simulink model "Identyfikacja"  (R2023b)
settings: Solver=FixedStepDiscrete  StartTime=0.0  StopTime=tend  RelTol=1e-3  EnableMultiTasking=on
values from neighbouring files (symbols this model uses):
  Tp = 0.01    [Init_Projekt.m]
settings Model: Creator=kszygenda  LastModifiedBy=Rafał
settings SolverCC: AlgebraicLoopSolver=TrustRegion
settings DataIOCC: LimitDataPoints=on  SaveFormat=Array  SignalLoggingSaveFormat=ModelDataLogs  ReturnWorkspaceOutputs=off
settings OptimizationCC: InitFltsAndDblsToZero=on  LifeSpan=inf
settings DebuggingCC: SaveWithParameterizedLinksMsg=none  UnderspecifiedInitializationDetection=Classic  MergeDetectMultiDrivingBlocksExec=none  SignalResolutionControl=TryResolveAllWithWarning  SolverPrmCheckMsg=warning  MultiTaskDSMMsg=warning  MultiTaskCondExecSysMsg=none  FcnCallInpInsideContextMsg=warning  UnconnectedInputMsg=warning  UnconnectedOutputMsg=warning  UnconnectedLineMsg=warning  SFUnexpectedBacktrackingDiag=warning  SFNoUnconditionalDefaultTransitionDiag=warning  SFExecutionAtInitializationDiag=none  ArithmeticOperatorsInVariantConditions=warning
settings HardwareCC: ProdBitPerPointer=32  ProdBitPerSizeT=32  ProdBitPerPtrDiffT=32  ProdLargestAtomicFloat=None  ProdIntDivRoundTo=Undefined  ProdEndianess=Unspecified  ProdWordSize=32  ProdHWDeviceType=32-bit Generic
settings ModelReferenceCC: PropagateSignalLabelsOutOfModel=off
settings CodeAppCC: StateflowObjectComments=on
settings GRTTargetCC: TargetFcnLib=ansi_tfl_tmw.mat  TargetLangStandard=C89/C90 (ANSI)  CombineOutputUpdateFcns=off  GRTInterface=on
settings ConfigComp: CovMetricSettings=dw  CovSaveCumulativeToWorkspaceVar=on  CovSaveSingleToWorkspaceVar=on

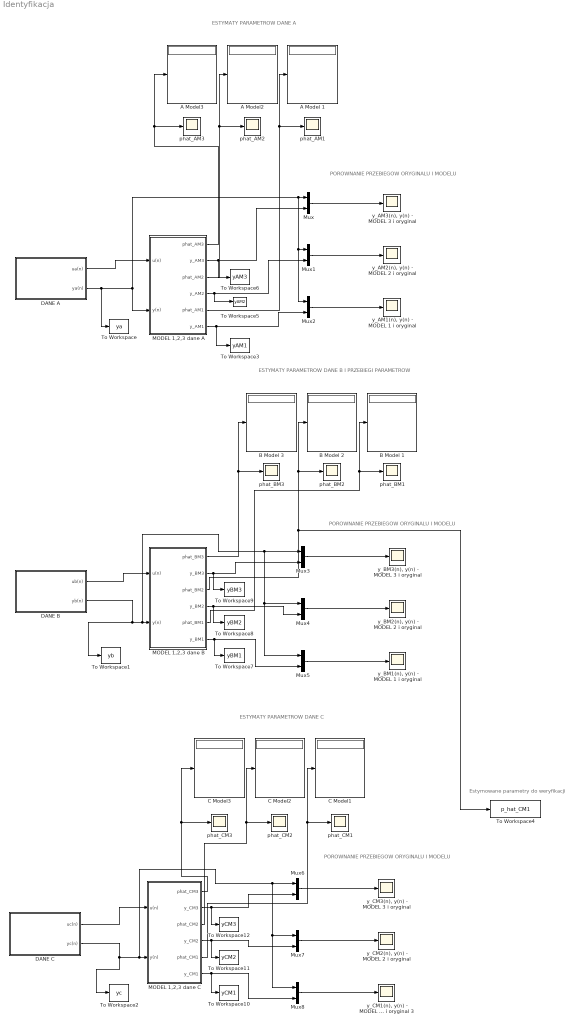
== system Identyfikacja ==
  note: Estymowane parametry do weryfikacji
  note: ESTYMATY PARAMETROW DANE A
  note: ESTYMATY PARAMETROW DANE B I PRZEBIEGI PARAMETROW
  note: ESTYMATY PARAMETROW DANE C
  note: POROWNANIE PRZEBIEGOW ORYGINALU I MODELU
  note: POROWNANIE PRZEBIEGOW ORYGINALU I MODELU
  note: POROWNANIE PRZEBIEGOW ORYGINALU I MODELU
  A Model 1 : Display
  A Model2 : Display
  A Model3 : Display
  B Model 1 : Display
  B Model 2 : Display
  B Model 3 : Display
  C Model1 : Display
  C Model2 : Display
  C Model3 : Display
  DANE A : Subsystem
  DANE B : Subsystem
  DANE C : Subsystem
  MODEL 1,2,3 dane A : Subsystem
  MODEL 1,2,3 dane B : Subsystem
  MODEL 1,2,3 dane C : Subsystem
  Mux{,1..8} (9 alike) : Mux  Inputs=2
  To Workspace : ToWorkspace  VariableName=ya  SampleTime=Tp
      settings: Save2DSignal=2-D array (concatenate along first dimension)
  To Workspace1 : ToWorkspace  VariableName=yb  SampleTime=Tp
      settings: Save2DSignal=2-D array (concatenate along first dimension)
  To Workspace10 : ToWorkspace  VariableName=yCM1  SampleTime=Tp
      settings: Save2DSignal=2-D array (concatenate along first dimension)
  To Workspace11 : ToWorkspace  VariableName=yCM2  SampleTime=Tp
      settings: Save2DSignal=2-D array (concatenate along first dimension)
  To Workspace12 : ToWorkspace  VariableName=yCM3  SampleTime=Tp
      settings: Save2DSignal=2-D array (concatenate along first dimension)
  To Workspace2 : ToWorkspace  VariableName=yc  SampleTime=Tp
      settings: Save2DSignal=2-D array (concatenate along first dimension)
  To Workspace3 : ToWorkspace  VariableName=yAM1  SampleTime=Tp
      settings: Save2DSignal=2-D array (concatenate along first dimension)
  To Workspace4 : ToWorkspace  VariableName=p_hat_CM1  SampleTime=Tp
      settings: Save2DSignal=2-D array (concatenate along first dimension)
  To Workspace5 : ToWorkspace  VariableName=yAM2  SampleTime=Tp
      settings: Save2DSignal=2-D array (concatenate along first dimension)
  To Workspace6 : ToWorkspace  VariableName=yAM3  SampleTime=Tp
      settings: Save2DSignal=2-D array (concatenate along first dimension)
  To Workspace7 : ToWorkspace  VariableName=yBM1  SampleTime=Tp
      settings: Save2DSignal=2-D array (concatenate along first dimension)
  To Workspace8 : ToWorkspace  VariableName=yBM2  SampleTime=Tp
      settings: Save2DSignal=2-D array (concatenate along first dimension)
  To Workspace9 : ToWorkspace  VariableName=yBM3  SampleTime=Tp
      settings: Save2DSignal=2-D array (concatenate along first dimension)
  phat_AM1 : Scope
  phat_AM2 : Scope
  phat_AM3 : Scope
  phat_BM1 : Scope
  phat_BM2 : Scope
  phat_BM3 : Scope
  phat_CM1 : Scope
  phat_CM2 : Scope
  phat_CM3 : Scope
  "y_AM1(n), y(n) - MODEL 1 i oryginal" : Scope
  "y_AM2(n), y(n) - MODEL 2 i oryginal " : Scope
  "y_AM3(n), y(n) - MODEL 3 i oryginal " : Scope
  "y_BM1(n), y(n) - MODEL 1 i oryginal" : Scope
  "y_BM2(n), y(n) - MODEL 2 i oryginal" : Scope
  "y_BM3(n), y(n) - MODEL 3 i oryginal" : Scope
  "y_CM1(n), y(n) - MODEL 1 i oryginal 3" : Scope
  "y_CM2(n), y(n) - MODEL 2 i oryginal" : Scope
  "y_CM3(n), y(n) - MODEL 3 i oryginal" : Scope
  wires:
  DANE C/1(uc(n)) -> MODEL 1,2,3 dane C/1(u(n))
  DANE C/2(yc(n)) -> To Workspace2/1, Mux6/1, Mux7/1, Mux8/1, MODEL 1,2,3 dane C/2(y(n))
  DANE B/1(ub(n)) -> MODEL 1,2,3 dane B/1(u(n))
  DANE B/2(yb(n)) -> To Workspace1/1, Mux3/1, Mux5/1, Mux4/1, MODEL 1,2,3 dane B/2(y(n))
  DANE A/1(ua(n)) -> MODEL 1,2,3 dane A/1(u(n))
  DANE A/2(ya(n)) -> To Workspace/1, Mux1/1, Mux2/1, Mux/1, MODEL 1,2,3 dane A/2(y(n))
  Mux/1 -> "y_AM3(n), y(n) - MODEL 3 i oryginal "/1
  MODEL 1,2,3 dane A/2(y_AM3) -> To Workspace6/1, Mux/2
  Mux1/1 -> "y_AM2(n), y(n) - MODEL 2 i oryginal "/1
  Mux2/1 -> "y_AM1(n), y(n) - MODEL 1 i oryginal"/1
  Mux3/1 -> "y_BM3(n), y(n) - MODEL 3 i oryginal"/1
  Mux5/1 -> "y_BM1(n), y(n) - MODEL 1 i oryginal"/1
  Mux4/1 -> "y_BM2(n), y(n) - MODEL 2 i oryginal"/1
  Mux6/1 -> "y_CM3(n), y(n) - MODEL 3 i oryginal"/1
  Mux8/1 -> "y_CM1(n), y(n) - MODEL 1 i oryginal 3"/1
  Mux7/1 -> "y_CM2(n), y(n) - MODEL 2 i oryginal"/1
  MODEL 1,2,3 dane A/4(y_AM2) -> Mux1/2, To Workspace5/1
  MODEL 1,2,3 dane A/6(y_AM1) -> Mux2/2, To Workspace3/1
  MODEL 1,2,3 dane C/2(y_CM3) -> To Workspace12/1, Mux6/2
  MODEL 1,2,3 dane C/4(y_CM2) -> To Workspace11/1, Mux7/2
  MODEL 1,2,3 dane C/6(y_CM1) -> To Workspace10/1, Mux8/2
  MODEL 1,2,3 dane B/2(y_BM3) -> To Workspace9/1, Mux3/2
  MODEL 1,2,3 dane B/4(y_BM2) -> To Workspace8/1, Mux4/2
  MODEL 1,2,3 dane B/6(y_BM1) -> To Workspace7/1, Mux5/2
  MODEL 1,2,3 dane A/1(phat_AM3) -> phat_AM3/1, A Model3/1
  MODEL 1,2,3 dane A/3(phat_AM2) -> phat_AM2/1, A Model2/1
  MODEL 1,2,3 dane A/5(phat_AM1) -> A Model 1/1, phat_AM1/1
  MODEL 1,2,3 dane B/1(phat_BM3) -> phat_BM3/1, B Model 3/1
  MODEL 1,2,3 dane B/3(phat_BM2) -> phat_BM2/1, B Model 2/1, To Workspace4/1
  MODEL 1,2,3 dane B/5(phat_BM1) -> B Model 1/1, phat_BM1/1
  MODEL 1,2,3 dane C/1(phat_CM3) -> phat_CM3/1, C Model3/1
  MODEL 1,2,3 dane C/3(phat_CM2) -> phat_CM2/1, C Model2/1
  MODEL 1,2,3 dane C/5(phat_CM1) -> phat_CM1/1, C Model1/1

== system Identyfikacja/DANE A ==
  Demux : Demux  Outputs=2
  From Workspace : FromWorkspace  VariableName=to_simA  SampleTime=Tp
  ua(n) : Outport
  ya(n) : Outport  Port=2
  wires:
  Demux/1 -> ua(n)/1
  From Workspace/1 -> Demux/1
  Demux/2 -> ya(n)/1

== system Identyfikacja/DANE B ==
  Demux : Demux  Outputs=2
  From Workspace : FromWorkspace  VariableName=to_simB  SampleTime=Tp
  ub(n) : Outport
  yb(n) : Outport  Port=2
  wires:
  Demux/1 -> ub(n)/1
  From Workspace/1 -> Demux/1
  Demux/2 -> yb(n)/1

== system Identyfikacja/DANE C ==
  Demux : Demux  Outputs=2
  From Workspace : FromWorkspace  VariableName=to_simC  SampleTime=Tp
  uc(n) : Outport
  yc(n) : Outport  Port=2
  wires:
  Demux/1 -> uc(n)/1
  From Workspace/1 -> Demux/1
  Demux/2 -> yc(n)/1

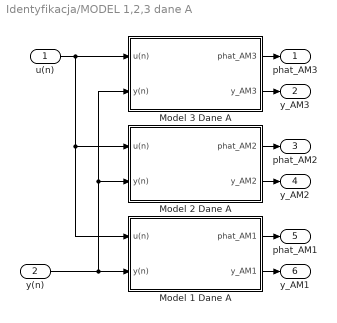
== system Identyfikacja/MODEL 1,2,3 dane A ==
  u(n) : Inport
  y(n) : Inport  Port=2
  Model 1 Dane A : Subsystem
  Model 2 Dane A : Subsystem
  Model 3 Dane A : Subsystem
  phat_AM3 : Outport
  y_AM3 : Outport  Port=2
  phat_AM2 : Outport  Port=3
  y_AM2 : Outport  Port=4
  phat_AM1 : Outport  Port=5
  y_AM1 : Outport  Port=6
  wires:
  Model 1 Dane A/1(phat_AM1) -> phat_AM1/1
  u(n)/1 -> Model 3 Dane A/1(u(n)), Model 2 Dane A/1(u(n)), Model 1 Dane A/1(u(n))
  Model 1 Dane A/2(y_AM1) -> y_AM1/1
  y(n)/1 -> Model 2 Dane A/2(y(n)), Model 3 Dane A/2(y(n)), Model 1 Dane A/2(y(n))
  Model 3 Dane A/1(phat_AM3) -> phat_AM3/1
  Model 3 Dane A/2(y_AM3) -> y_AM3/1
  Model 2 Dane A/2(y_AM2) -> y_AM2/1
  Model 2 Dane A/1(phat_AM2) -> phat_AM2/1

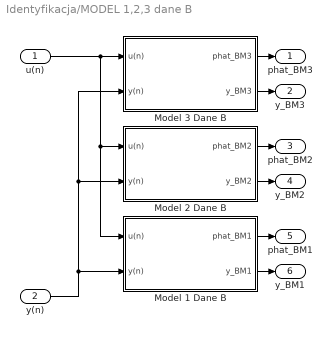
== system Identyfikacja/MODEL 1,2,3 dane B ==
  u(n) : Inport
  y(n) : Inport  Port=2
  Model 1 Dane B : Subsystem
  Model 2 Dane B : Subsystem
  Model 3 Dane B : Subsystem
  phat_BM3 : Outport
  y_BM3 : Outport  Port=2
  phat_BM2 : Outport  Port=3
  y_BM2 : Outport  Port=4
  phat_BM1 : Outport  Port=5
  y_BM1 : Outport  Port=6
  wires:
  Model 3 Dane B/1(phat_BM3) -> phat_BM3/1
  u(n)/1 -> Model 3 Dane B/1(u(n)), Model 2 Dane B/1(u(n)), Model 1 Dane B/1(u(n))
  Model 1 Dane B/1(phat_BM1) -> phat_BM1/1
  Model 3 Dane B/2(y_BM3) -> y_BM3/1
  y(n)/1 -> Model 1 Dane B/2(y(n)), Model 2 Dane B/2(y(n)), Model 3 Dane B/2(y(n))
  Model 2 Dane B/2(y_BM2) -> y_BM2/1
  Model 1 Dane B/2(y_BM1) -> y_BM1/1
  Model 2 Dane B/1(phat_BM2) -> phat_BM2/1

== system Identyfikacja/MODEL 1,2,3 dane C ==
  u(n) : Inport
  y(n) : Inport  Port=2
  Model 1 Dane C : Subsystem
  Model 2 Dane C : Subsystem
  Model 3 Dane C : Subsystem
  phat_CM3 : Outport
  y_CM3 : Outport  Port=2
  phat_CM2 : Outport  Port=3
  y_CM2 : Outport  Port=4
  phat_CM1 : Outport  Port=5
  y_CM1 : Outport  Port=6
  wires:
  u(n)/1 -> Model 3 Dane C/1(u(n)), Model 2 Dane C/1(u(n)), Model 1 Dane C/1(u(n))
  Model 2 Dane C/2(y_CM2) -> y_CM2/1
  Model 3 Dane C/2(y_CM3) -> y_CM3/1
  Model 3 Dane C/1(phat_CM3) -> phat_CM3/1
  Model 1 Dane C/2(y_CM1) -> y_CM1/1
  Model 2 Dane C/1(phat_CM2) -> phat_CM2/1
  Model 1 Dane C/1(phat_CM1) -> phat_CM1/1
  y(n)/1 -> Model 1 Dane C/2(y(n)), Model 2 Dane C/2(y(n)), Model 3 Dane C/2(y(n))

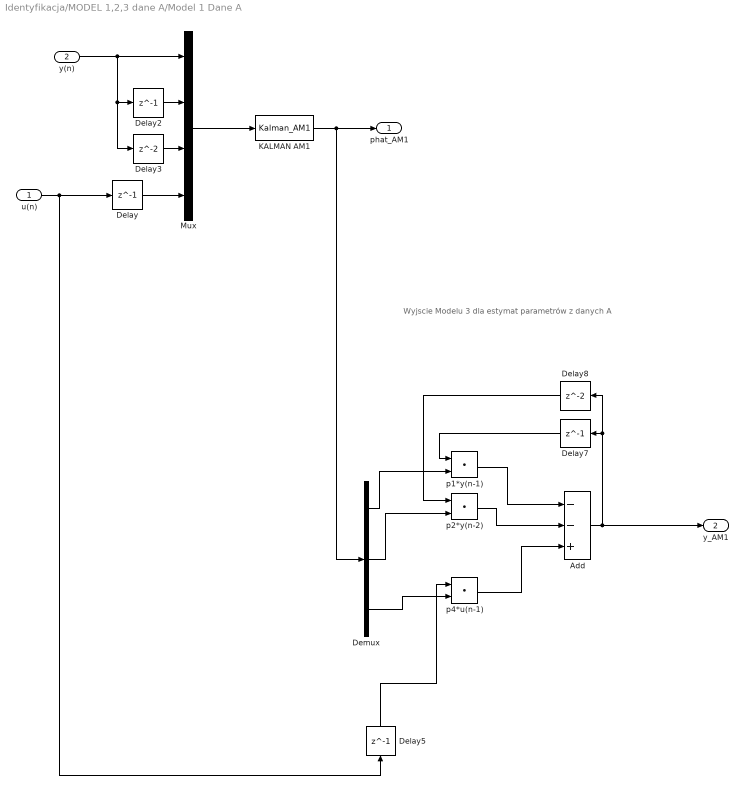
== system Identyfikacja/MODEL 1,2,3 dane A/Model 1 Dane A ==
  note: Wyjscie Modelu 3 dla estymat parametrów z danych A
  u(n) : Inport
  y(n) : Inport  Port=2
  Add : Sum  Inputs=--+
  Delay{,2,5,7} (4 alike) : Delay  DelayLength=1  InitialCondition=0  SampleTime=Tp
  Delay3 : Delay  InitialCondition=0  SampleTime=Tp
  Delay8 : Delay  InitialCondition=0  SampleTime=Tp
  Demux : Demux  Outputs=3
  KALMAN AM1 : MATLABFcn  MATLABFcn=Kalman_AM1  OutputDimensions=3
  Mux : Mux
  p1*y(n-1) : DotProduct  OutDataTypeStr=Inherit: Inherit via internal rule
  p2*y(n-2) : DotProduct  OutDataTypeStr=Inherit: Inherit via internal rule
  p4*u(n-1) : DotProduct  OutDataTypeStr=Inherit: Inherit via internal rule
  phat_AM1 : Outport
  y_AM1 : Outport  Port=2
  wires:
  y(n)/1 -> Mux/1, Delay3/1, Delay2/1
  Mux/1 -> KALMAN AM1/1
  KALMAN AM1/1 -> Demux/1, phat_AM1/1
  p1*y(n-1)/1 -> Add/1
  Demux/2 -> p2*y(n-2)/2
  Delay8/1 -> p2*y(n-2)/1
  p2*y(n-2)/1 -> Add/2
  Delay5/1 -> p4*u(n-1)/1
  Delay7/1 -> p1*y(n-1)/1
  Demux/1 -> p1*y(n-1)/2
  u(n)/1 -> Delay/1, Delay5/1
  Demux/3 -> p4*u(n-1)/2
  Add/1 -> y_AM1/1, Delay8/1, Delay7/1
  p4*u(n-1)/1 -> Add/3
  Delay2/1 -> Mux/2
  Delay3/1 -> Mux/3
  Delay/1 -> Mux/4

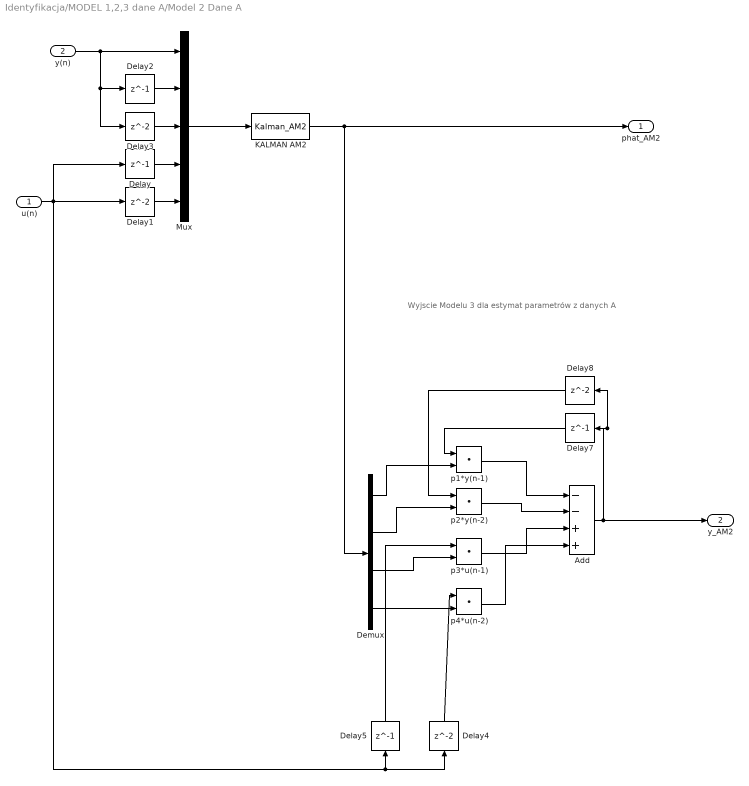
== system Identyfikacja/MODEL 1,2,3 dane A/Model 2 Dane A ==
  note: Wyjscie Modelu 3 dla estymat parametrów z danych A
  u(n) : Inport
  y(n) : Inport  Port=2
  Add : Sum  Inputs=--++
  Delay{,2,5,7} (4 alike) : Delay  DelayLength=1  InitialCondition=0  SampleTime=Tp
  Delay{1,3..4,8} (4 alike) : Delay  InitialCondition=0  SampleTime=Tp
  Demux : Demux
  KALMAN AM2 : MATLABFcn  MATLABFcn=Kalman_AM2  OutputDimensions=4
  Mux : Mux  Inputs=5
  p1*y(n-1) : DotProduct  OutDataTypeStr=Inherit: Inherit via internal rule
  p2*y(n-2) : DotProduct  OutDataTypeStr=Inherit: Inherit via internal rule
  p3*u(n-1) : DotProduct  OutDataTypeStr=Inherit: Inherit via internal rule
  p4*u(n-2) : DotProduct  OutDataTypeStr=Inherit: Inherit via internal rule
  phat_AM2 : Outport
  y_AM2 : Outport  Port=2
  wires:
  y(n)/1 -> Mux/1, Delay3/1, Delay2/1
  Delay5/1 -> p3*u(n-1)/1
  p1*y(n-1)/1 -> Add/1
  Demux/2 -> p2*y(n-2)/2
  p2*y(n-2)/1 -> Add/2
  Delay7/1 -> p1*y(n-1)/1
  Delay4/1 -> p4*u(n-2)/1
  Delay/1 -> Mux/4
  KALMAN AM2/1 -> Demux/1, phat_AM2/1
  Demux/4 -> p4*u(n-2)/2
  Add/1 -> Delay8/1, Delay7/1, y_AM2/1
  Delay8/1 -> p2*y(n-2)/1
  Delay3/1 -> Mux/3
  u(n)/1 -> Delay/1, Delay1/1, Delay4/1, Delay5/1
  Delay2/1 -> Mux/2
  Demux/3 -> p3*u(n-1)/2
  p4*u(n-2)/1 -> Add/4
  Delay1/1 -> Mux/5
  p3*u(n-1)/1 -> Add/3
  Mux/1 -> KALMAN AM2/1
  Demux/1 -> p1*y(n-1)/2

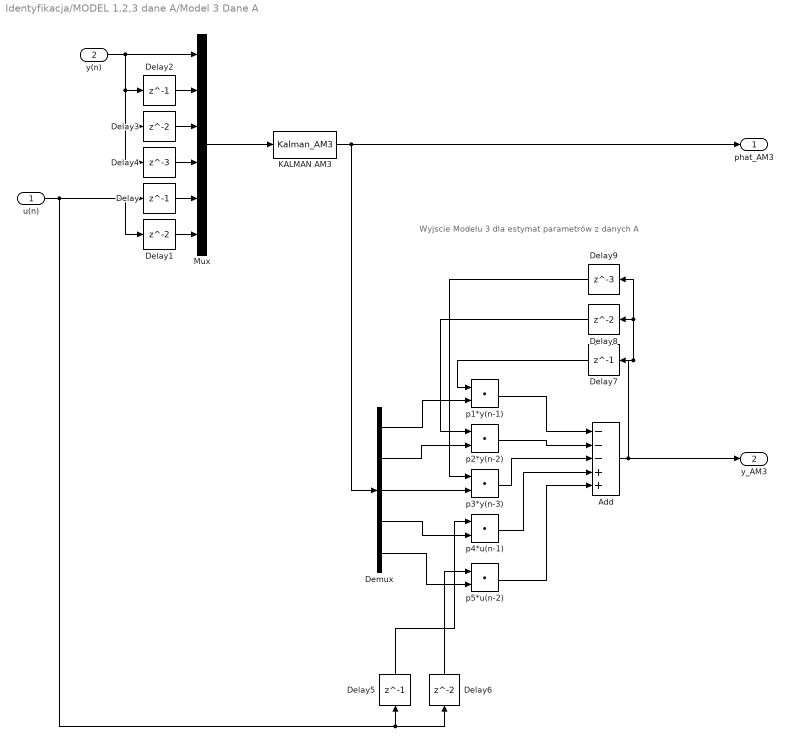
== system Identyfikacja/MODEL 1,2,3 dane A/Model 3 Dane A ==
  note: Wyjscie Modelu 3 dla estymat parametrów z danych A
  u(n) : Inport
  y(n) : Inport  Port=2
  Add : Sum  Inputs=---++
  Delay{,2,5,7} (4 alike) : Delay  DelayLength=1  InitialCondition=0  SampleTime=Tp
  Delay{1,3,6,8} (4 alike) : Delay  InitialCondition=0  SampleTime=Tp
  Delay4 : Delay  DelayLength=3  InitialCondition=0  SampleTime=Tp
  Delay9 : Delay  DelayLength=3  InitialCondition=0  SampleTime=Tp
  Demux : Demux  Outputs=5
  KALMAN AM3 : MATLABFcn  MATLABFcn=Kalman_AM3  OutputDimensions=5
  Mux : Mux  Inputs=6
  p1*y(n-1) : DotProduct  OutDataTypeStr=Inherit: Inherit via internal rule
  p2*y(n-2) : DotProduct  OutDataTypeStr=Inherit: Inherit via internal rule
  p3*y(n-3) : DotProduct  OutDataTypeStr=Inherit: Inherit via internal rule
  p4*u(n-1) : DotProduct  OutDataTypeStr=Inherit: Inherit via internal rule
  p5*u(n-2) : DotProduct  OutDataTypeStr=Inherit: Inherit via internal rule
  phat_AM3 : Outport
  y_AM3 : Outport  Port=2
  wires:
  KALMAN AM3/1 -> Demux/1, phat_AM3/1
  y(n)/1 -> Mux/1, Delay4/1, Delay3/1, Delay2/1
  Mux/1 -> KALMAN AM3/1
  Add/1 -> Delay9/1, Delay8/1, Delay7/1, y_AM3/1
  Demux/1 -> p1*y(n-1)/2
  Demux/2 -> p2*y(n-2)/2
  Demux/5 -> p5*u(n-2)/2
  Demux/4 -> p4*u(n-1)/2
  Demux/3 -> p3*y(n-3)/2
  u(n)/1 -> Delay6/1, Delay5/1, Delay1/1, Delay/1
  Delay5/1 -> p4*u(n-1)/1
  Delay6/1 -> p5*u(n-2)/1
  p5*u(n-2)/1 -> Add/5
  p4*u(n-1)/1 -> Add/4
  p3*y(n-3)/1 -> Add/3
  p2*y(n-2)/1 -> Add/2
  p1*y(n-1)/1 -> Add/1
  Delay7/1 -> p1*y(n-1)/1
  Delay8/1 -> p2*y(n-2)/1
  Delay9/1 -> p3*y(n-3)/1
  Delay4/1 -> Mux/4
  Delay3/1 -> Mux/3
  Delay2/1 -> Mux/2
  Delay1/1 -> Mux/6
  Delay/1 -> Mux/5

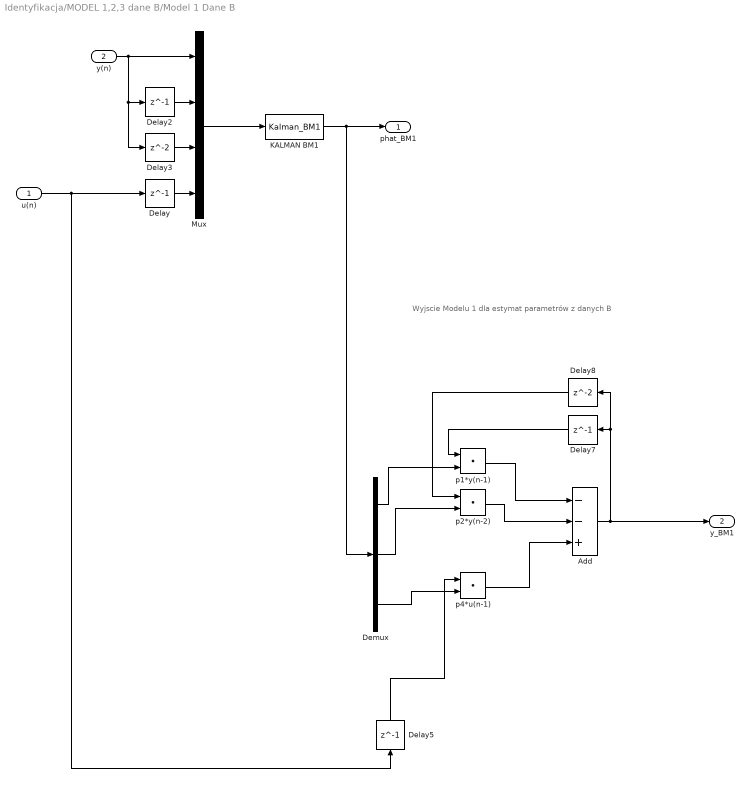
== system Identyfikacja/MODEL 1,2,3 dane B/Model 1 Dane B ==
  note: Wyjscie Modelu 1 dla estymat parametrów z danych B
  u(n) : Inport
  y(n) : Inport  Port=2
  Add : Sum  Inputs=--+
  Delay{,2,5,7} (4 alike) : Delay  DelayLength=1  InitialCondition=0  SampleTime=Tp
  Delay3 : Delay  InitialCondition=0  SampleTime=Tp
  Delay8 : Delay  InitialCondition=0  SampleTime=Tp
  Demux : Demux  Outputs=3
  KALMAN BM1 : MATLABFcn  MATLABFcn=Kalman_BM1  OutputDimensions=3
  Mux : Mux
  p1*y(n-1) : DotProduct  OutDataTypeStr=Inherit: Inherit via internal rule
  p2*y(n-2) : DotProduct  OutDataTypeStr=Inherit: Inherit via internal rule
  p4*u(n-1) : DotProduct  OutDataTypeStr=Inherit: Inherit via internal rule
  phat_BM1 : Outport
  y_BM1 : Outport  Port=2
  wires:
  y(n)/1 -> Mux/1, Delay3/1, Delay2/1
  Mux/1 -> KALMAN BM1/1
  KALMAN BM1/1 -> Demux/1, phat_BM1/1
  p1*y(n-1)/1 -> Add/1
  Demux/2 -> p2*y(n-2)/2
  Delay8/1 -> p2*y(n-2)/1
  p2*y(n-2)/1 -> Add/2
  Delay5/1 -> p4*u(n-1)/1
  Delay7/1 -> p1*y(n-1)/1
  Demux/1 -> p1*y(n-1)/2
  u(n)/1 -> Delay5/1, Delay/1
  Demux/3 -> p4*u(n-1)/2
  Add/1 -> y_BM1/1, Delay8/1, Delay7/1
  p4*u(n-1)/1 -> Add/3
  Delay3/1 -> Mux/3
  Delay2/1 -> Mux/2
  Delay/1 -> Mux/4

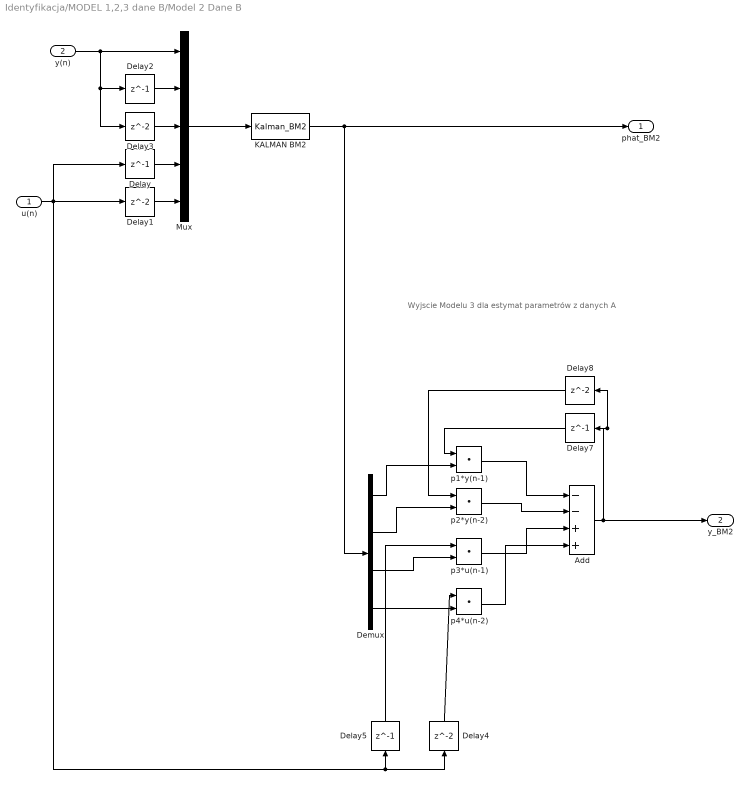
== system Identyfikacja/MODEL 1,2,3 dane B/Model 2 Dane B ==
  note: Wyjscie Modelu 3 dla estymat parametrów z danych A
  u(n) : Inport
  y(n) : Inport  Port=2
  Add : Sum  Inputs=--++
  Delay{,2,5,7} (4 alike) : Delay  DelayLength=1  InitialCondition=0  SampleTime=Tp
  Delay{1,3..4,8} (4 alike) : Delay  InitialCondition=0  SampleTime=Tp
  Demux : Demux
  KALMAN BM2 : MATLABFcn  MATLABFcn=Kalman_BM2  OutputDimensions=4
  Mux : Mux  Inputs=5
  p1*y(n-1) : DotProduct  OutDataTypeStr=Inherit: Inherit via internal rule
  p2*y(n-2) : DotProduct  OutDataTypeStr=Inherit: Inherit via internal rule
  p3*u(n-1) : DotProduct  OutDataTypeStr=Inherit: Inherit via internal rule
  p4*u(n-2) : DotProduct  OutDataTypeStr=Inherit: Inherit via internal rule
  phat_BM2 : Outport
  y_BM2 : Outport  Port=2
  wires:
  y(n)/1 -> Mux/1, Delay3/1, Delay2/1
  Mux/1 -> KALMAN BM2/1
  u(n)/1 -> Delay/1, Delay1/1, Delay4/1, Delay5/1
  Delay8/1 -> p2*y(n-2)/1
  Add/1 -> Delay8/1, Delay7/1, y_BM2/1
  Demux/1 -> p1*y(n-1)/2
  Delay7/1 -> p1*y(n-1)/1
  Delay5/1 -> p3*u(n-1)/1
  KALMAN BM2/1 -> Demux/1, phat_BM2/1
  p2*y(n-2)/1 -> Add/2
  Demux/2 -> p2*y(n-2)/2
  p1*y(n-1)/1 -> Add/1
  Delay3/1 -> Mux/3
  Delay2/1 -> Mux/2
  Delay/1 -> Mux/4
  Delay1/1 -> Mux/5
  Demux/3 -> p3*u(n-1)/2
  p3*u(n-1)/1 -> Add/3
  Delay4/1 -> p4*u(n-2)/1
  Demux/4 -> p4*u(n-2)/2
  p4*u(n-2)/1 -> Add/4

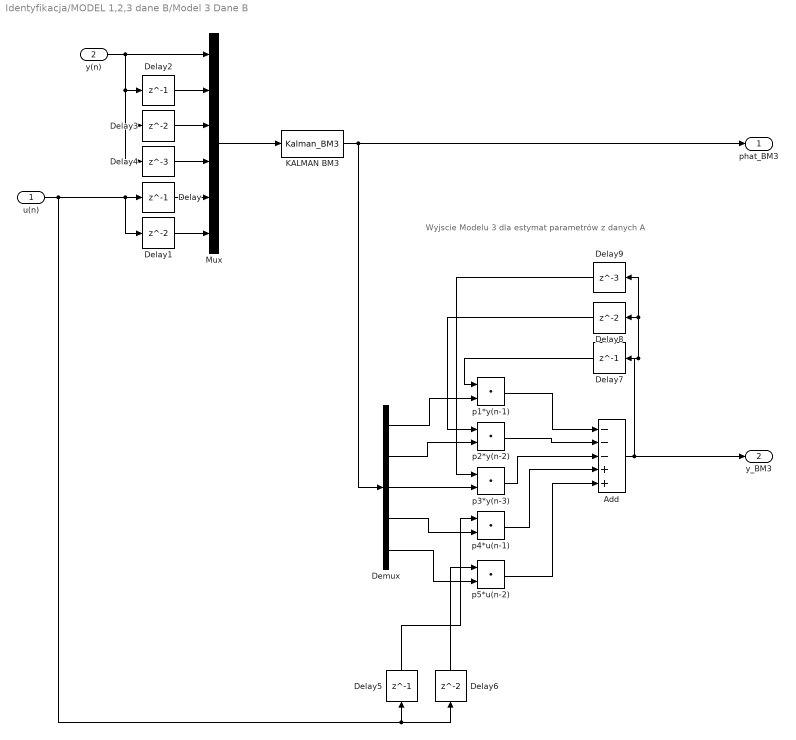
== system Identyfikacja/MODEL 1,2,3 dane B/Model 3 Dane B ==
  note: Wyjscie Modelu 3 dla estymat parametrów z danych A
  u(n) : Inport
  y(n) : Inport  Port=2
  Add : Sum  Inputs=---++
  Delay{,2,5,7} (4 alike) : Delay  DelayLength=1  InitialCondition=0  SampleTime=Tp
  Delay{1,3,6,8} (4 alike) : Delay  InitialCondition=0  SampleTime=Tp
  Delay4 : Delay  DelayLength=3  InitialCondition=0  SampleTime=Tp
  Delay9 : Delay  DelayLength=3  InitialCondition=0  SampleTime=Tp
  Demux : Demux  Outputs=5
  KALMAN BM3 : MATLABFcn  MATLABFcn=Kalman_BM3  OutputDimensions=5
  Mux : Mux  Inputs=6
  p1*y(n-1) : DotProduct  OutDataTypeStr=Inherit: Inherit via internal rule
  p2*y(n-2) : DotProduct  OutDataTypeStr=Inherit: Inherit via internal rule
  p3*y(n-3) : DotProduct  OutDataTypeStr=Inherit: Inherit via internal rule
  p4*u(n-1) : DotProduct  OutDataTypeStr=Inherit: Inherit via internal rule
  p5*u(n-2) : DotProduct  OutDataTypeStr=Inherit: Inherit via internal rule
  phat_BM3 : Outport
  y_BM3 : Outport  Port=2
  wires:
  KALMAN BM3/1 -> Demux/1, phat_BM3/1
  y(n)/1 -> Mux/1, Delay4/1, Delay3/1, Delay2/1
  Mux/1 -> KALMAN BM3/1
  Add/1 -> Delay9/1, Delay8/1, Delay7/1, y_BM3/1
  Demux/1 -> p1*y(n-1)/2
  Demux/2 -> p2*y(n-2)/2
  Demux/5 -> p5*u(n-2)/2
  Demux/4 -> p4*u(n-1)/2
  Demux/3 -> p3*y(n-3)/2
  u(n)/1 -> Delay6/1, Delay5/1, Delay1/1, Delay/1
  Delay5/1 -> p4*u(n-1)/1
  Delay6/1 -> p5*u(n-2)/1
  p5*u(n-2)/1 -> Add/5
  p4*u(n-1)/1 -> Add/4
  p3*y(n-3)/1 -> Add/3
  p2*y(n-2)/1 -> Add/2
  p1*y(n-1)/1 -> Add/1
  Delay7/1 -> p1*y(n-1)/1
  Delay8/1 -> p2*y(n-2)/1
  Delay9/1 -> p3*y(n-3)/1
  Delay4/1 -> Mux/4
  Delay3/1 -> Mux/3
  Delay2/1 -> Mux/2
  Delay/1 -> Mux/5
  Delay1/1 -> Mux/6

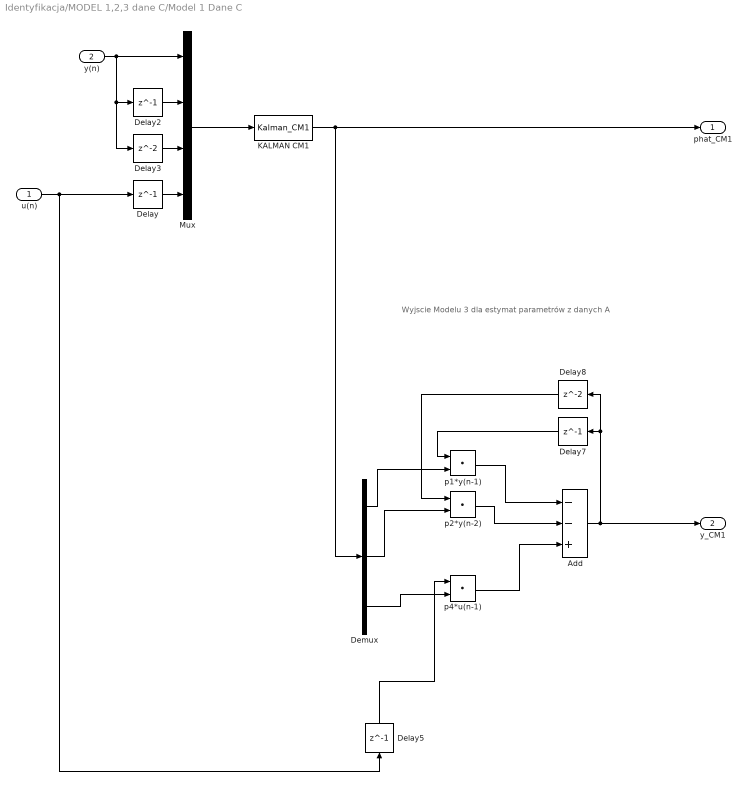
== system Identyfikacja/MODEL 1,2,3 dane C/Model 1 Dane C ==
  note: Wyjscie Modelu 3 dla estymat parametrów z danych A
  u(n) : Inport
  y(n) : Inport  Port=2
  Add : Sum  Inputs=--+
  Delay{,2,5,7} (4 alike) : Delay  DelayLength=1  InitialCondition=0  SampleTime=Tp
  Delay3 : Delay  InitialCondition=0  SampleTime=Tp
  Delay8 : Delay  InitialCondition=0  SampleTime=Tp
  Demux : Demux  Outputs=3
  KALMAN CM1 : MATLABFcn  MATLABFcn=Kalman_CM1  OutputDimensions=3
  Mux : Mux
  p1*y(n-1) : DotProduct  OutDataTypeStr=Inherit: Inherit via internal rule
  p2*y(n-2) : DotProduct  OutDataTypeStr=Inherit: Inherit via internal rule
  p4*u(n-1) : DotProduct  OutDataTypeStr=Inherit: Inherit via internal rule
  phat_CM1 : Outport
  y_CM1 : Outport  Port=2
  wires:
  y(n)/1 -> Mux/1, Delay3/1, Delay2/1
  Mux/1 -> KALMAN CM1/1
  KALMAN CM1/1 -> Demux/1, phat_CM1/1
  p1*y(n-1)/1 -> Add/1
  Demux/2 -> p2*y(n-2)/2
  Delay8/1 -> p2*y(n-2)/1
  p2*y(n-2)/1 -> Add/2
  Delay5/1 -> p4*u(n-1)/1
  Delay7/1 -> p1*y(n-1)/1
  Demux/1 -> p1*y(n-1)/2
  u(n)/1 -> Delay5/1, Delay/1
  Demux/3 -> p4*u(n-1)/2
  Add/1 -> y_CM1/1, Delay8/1, Delay7/1
  p4*u(n-1)/1 -> Add/3
  Delay3/1 -> Mux/3
  Delay2/1 -> Mux/2
  Delay/1 -> Mux/4

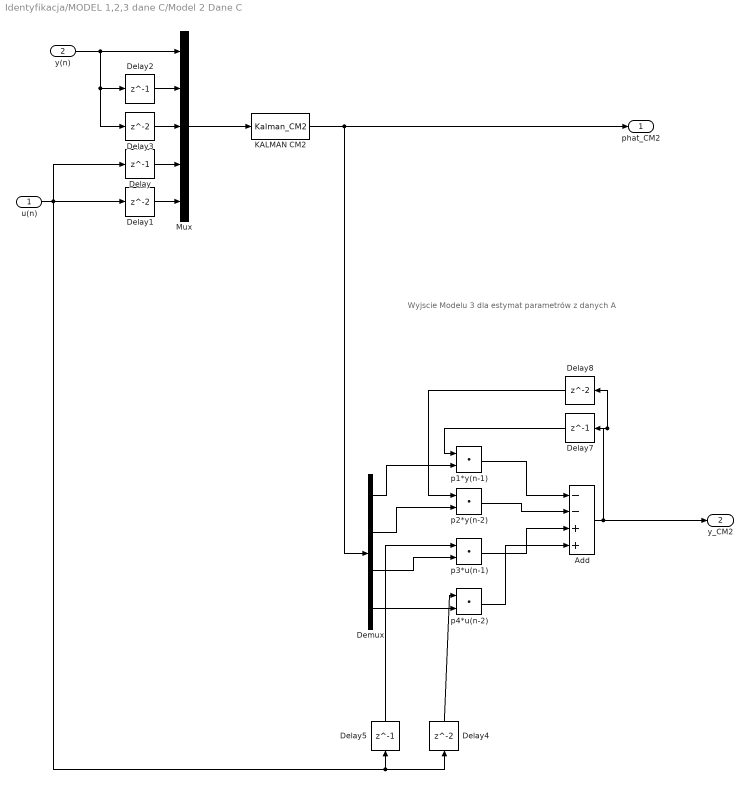
== system Identyfikacja/MODEL 1,2,3 dane C/Model 2 Dane C ==
  note: Wyjscie Modelu 3 dla estymat parametrów z danych A
  u(n) : Inport
  y(n) : Inport  Port=2
  Add : Sum  Inputs=--++
  Delay{,2,5,7} (4 alike) : Delay  DelayLength=1  InitialCondition=0  SampleTime=Tp
  Delay{1,3..4,8} (4 alike) : Delay  InitialCondition=0  SampleTime=Tp
  Demux : Demux
  KALMAN CM2 : MATLABFcn  MATLABFcn=Kalman_CM2  OutputDimensions=4
  Mux : Mux  Inputs=5
  p1*y(n-1) : DotProduct  OutDataTypeStr=Inherit: Inherit via internal rule
  p2*y(n-2) : DotProduct  OutDataTypeStr=Inherit: Inherit via internal rule
  p3*u(n-1) : DotProduct  OutDataTypeStr=Inherit: Inherit via internal rule
  p4*u(n-2) : DotProduct  OutDataTypeStr=Inherit: Inherit via internal rule
  phat_CM2 : Outport
  y_CM2 : Outport  Port=2
  wires:
  y(n)/1 -> Mux/1, Delay3/1, Delay2/1
  Delay5/1 -> p3*u(n-1)/1
  p1*y(n-1)/1 -> Add/1
  Demux/2 -> p2*y(n-2)/2
  p2*y(n-2)/1 -> Add/2
  Delay7/1 -> p1*y(n-1)/1
  Delay4/1 -> p4*u(n-2)/1
  Delay/1 -> Mux/4
  KALMAN CM2/1 -> Demux/1, phat_CM2/1
  Demux/4 -> p4*u(n-2)/2
  Add/1 -> Delay8/1, Delay7/1, y_CM2/1
  Delay8/1 -> p2*y(n-2)/1
  Delay3/1 -> Mux/3
  u(n)/1 -> Delay/1, Delay1/1, Delay4/1, Delay5/1
  Delay2/1 -> Mux/2
  Demux/3 -> p3*u(n-1)/2
  p4*u(n-2)/1 -> Add/4
  Delay1/1 -> Mux/5
  p3*u(n-1)/1 -> Add/3
  Mux/1 -> KALMAN CM2/1
  Demux/1 -> p1*y(n-1)/2

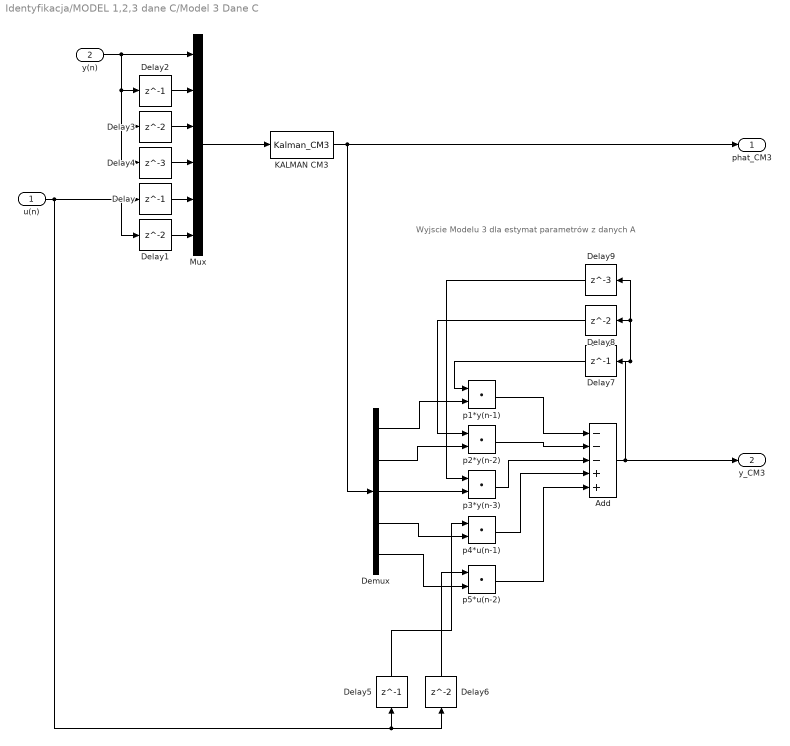
== system Identyfikacja/MODEL 1,2,3 dane C/Model 3 Dane C ==
  note: Wyjscie Modelu 3 dla estymat parametrów z danych A
  u(n) : Inport
  y(n) : Inport  Port=2
  Add : Sum  Inputs=---++
  Delay{,2,5,7} (4 alike) : Delay  DelayLength=1  InitialCondition=0  SampleTime=Tp
  Delay{1,3,6,8} (4 alike) : Delay  InitialCondition=0  SampleTime=Tp
  Delay4 : Delay  DelayLength=3  InitialCondition=0  SampleTime=Tp
  Delay9 : Delay  DelayLength=3  InitialCondition=0  SampleTime=Tp
  Demux : Demux  Outputs=5
  KALMAN CM3 : MATLABFcn  MATLABFcn=Kalman_CM3  OutputDimensions=5
  Mux : Mux  Inputs=6
  p1*y(n-1) : DotProduct  OutDataTypeStr=Inherit: Inherit via internal rule
  p2*y(n-2) : DotProduct  OutDataTypeStr=Inherit: Inherit via internal rule
  p3*y(n-3) : DotProduct  OutDataTypeStr=Inherit: Inherit via internal rule
  p4*u(n-1) : DotProduct  OutDataTypeStr=Inherit: Inherit via internal rule
  p5*u(n-2) : DotProduct  OutDataTypeStr=Inherit: Inherit via internal rule
  phat_CM3 : Outport
  y_CM3 : Outport  Port=2
  wires:
  KALMAN CM3/1 -> Demux/1, phat_CM3/1
  y(n)/1 -> Mux/1, Delay4/1, Delay3/1, Delay2/1
  Mux/1 -> KALMAN CM3/1
  Add/1 -> Delay9/1, Delay8/1, Delay7/1, y_CM3/1
  Demux/1 -> p1*y(n-1)/2
  Demux/2 -> p2*y(n-2)/2
  Demux/5 -> p5*u(n-2)/2
  Demux/4 -> p4*u(n-1)/2
  Demux/3 -> p3*y(n-3)/2
  u(n)/1 -> Delay6/1, Delay5/1, Delay1/1, Delay/1
  Delay5/1 -> p4*u(n-1)/1
  Delay6/1 -> p5*u(n-2)/1
  p5*u(n-2)/1 -> Add/5
  p4*u(n-1)/1 -> Add/4
  p3*y(n-3)/1 -> Add/3
  p2*y(n-2)/1 -> Add/2
  p1*y(n-1)/1 -> Add/1
  Delay7/1 -> p1*y(n-1)/1
  Delay8/1 -> p2*y(n-2)/1
  Delay9/1 -> p3*y(n-3)/1
  Delay4/1 -> Mux/4
  Delay3/1 -> Mux/3
  Delay2/1 -> Mux/2
  Delay1/1 -> Mux/6
  Delay/1 -> Mux/5
